simulink model "Adaptive_SMC"  (R2017b)
settings: Solver=ode45  StartTime=0.0  StopTime=20  RelTol=1e-3  EnableMultiTasking=on
settings Model: Creator=rushik  LastModifiedBy=thapa
settings SolverCC: MaxConsecutiveMinStep=5  ZeroCrossControl=EnableAll
settings DataIOCC: SaveOutput=off  SaveTime=off
settings OptimizationCC: LifeSpan=inf
settings DebuggingCC: SFUnexpectedBacktrackingDiag=warning  SFNoUnconditionalDefaultTransitionDiag=warning  SFExecutionAtInitializationDiag=none
settings ModelReferenceCC: ModelReferenceMinAlgLoopOccurrences=on
settings CodeAppCC: StateflowObjectComments=on
settings GRTTargetCC: TargetLangStandard=C89/C90 (ANSI)  CombineOutputUpdateFcns=off
settings ConfigComp: CovMetricSettings=dw  CovHtmlReporting=on  CovSaveCumulativeToWorkspaceVar=on  CovSaveSingleToWorkspaceVar=on  CovExternalEMLEnable=off

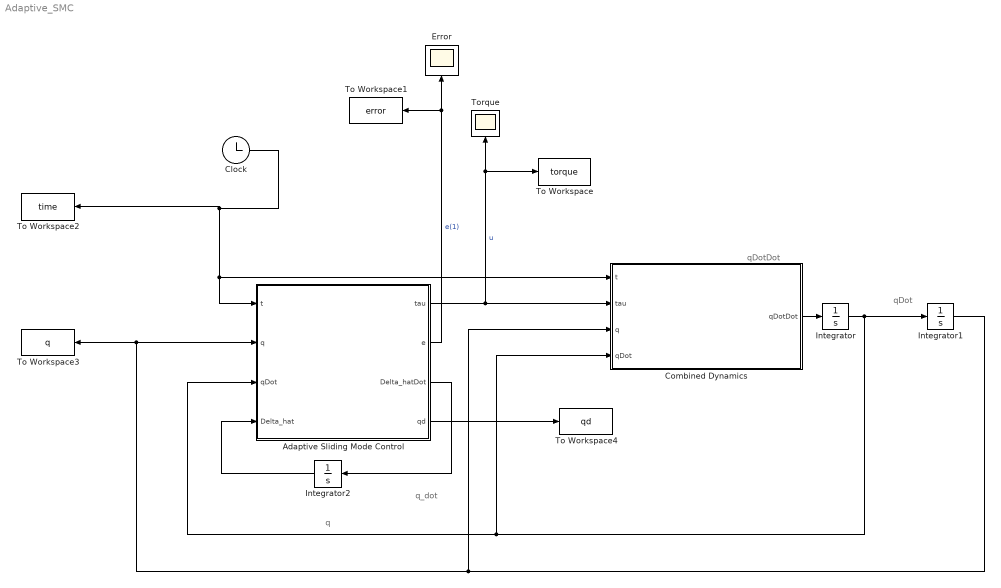
== system Adaptive_SMC ==
  note: q_dot
  note: q
  note: qDot
  note: qDotDot
  "Adaptive Sliding Mode Control " : MATLAB Function  TreatAsAtomicUnit=on
  Clock : Clock
      settings: Decimation=100
  "Combined Dynamics " : MATLAB Function  TreatAsAtomicUnit=on
  "Error " : Scope
  Integrator : Integrator  InitialCondition=[0;0;0;0;0;0;0;pi/2]  IgnoreLimit=on
  Integrator1 : Integrator  InitialCondition=[0;0;0;0;0;0;0;0]
  Integrator2 : Integrator  InitialCondition=[0;0;0;0;0;0;0;0]  IgnoreLimit=on
  To Workspace : ToWorkspace  VariableName=torque  SampleTime=-1
  To Workspace1 : ToWorkspace  VariableName=error  SampleTime=-1
  To Workspace2 : ToWorkspace  VariableName=time  SampleTime=-1
  To Workspace3 : ToWorkspace  VariableName=q  SampleTime=-1
  To Workspace4 : ToWorkspace  VariableName=qd  SampleTime=-1
  "Torque " : Scope
  wires:
  "Adaptive Sliding Mode Control "/1(tau) -> "Torque "/1, To Workspace/1, "Combined Dynamics "/2(tau)  "u"
  "Combined Dynamics "/1(qDotDot) -> Integrator/1
  Clock/1 -> "Adaptive Sliding Mode Control "/1(t), "Combined Dynamics "/1(t), To Workspace2/1
  "Adaptive Sliding Mode Control "/2(e) -> To Workspace1/1, "Error "/1  "e(1)"
  "Adaptive Sliding Mode Control "/3(Delta_hatDot) -> Integrator2/1
  Integrator2/1 -> "Adaptive Sliding Mode Control "/4(Delta_hat)
  Integrator/1 -> Integrator1/1, "Combined Dynamics "/4(qDot), "Adaptive Sliding Mode Control "/3(qDot)
  Integrator1/1 -> "Combined Dynamics "/3(q), To Workspace3/1, "Adaptive Sliding Mode Control "/2(q)
  "Adaptive Sliding Mode Control "/4(qd) -> To Workspace4/1

== matlab function Adaptive_SMC/Combined Dynamics  ==
  data: t input; tau input; qDotDot output; q input; qDot input
% Robot manipulator dynamics.
function qDotDot  = Aerial_Manipulator_dynamics(t, tau, q, qDot)

% q1 = q(1); q2 = q(2); % Joint angles
% q1_dot = q_dot(1); q2_dot = q_dot(2); % Joint angular velocities

x = q(1); 
y = q(2);
z = q(3);
phi = q(4);
theta = q(5);
psi = q(6); 
n1 = q(7);
n2 = q(8);

x_dot = qDot(1);
y_dot = qDot(2);
z_dot = qDot(3);
phi_dot = qDot(4);
theta_dot = qDot(5); 
psi_dot = qDot(6);
n1_dot = qDot(7);
n2_dot = qDot(8);

qd = [0 0 6 0 0 0 .5 .5]';
qdDot = [0 0 0 0 0 0 0 0]';
qdDotDot = [0 0 0 0 0 0 0 0]';

lamda = eye(8,8);
e = q - qd; 
eDot = qDot - qdDot;
s = eDot + lamda*e;
qrDot = qdDot-lamda*e;
qrDotDot = qdDotDot - lamda*eDot;

m_b = 2; 
Ixx = 1.24; 
Iyy = 1.24;
Izz = 2.48; 

m_1 = 0.049 ; 
Ix1 = 0.0011; 
Iy1 = Ix1; 
Iz1 = 0;
l1 = 0.015; 
l2 = 0.005;

Ix2 = 1.25/10000; 
Iy2 = Ix2; 
Iz2 = 0; 

m_2 = 0.05 ; 

p_b = [x y z]'; %postion of UAV with respect to inertial frame
p_b_dot = [x_dot y_dot z_dot]';
% An_b = [psi theta phi]'; %Euler angles used: yaw pitch roll 
% An_dot = [psi_dot theta_dot phi_dot]';
% n_b = [n1 n2]';  % joint angles 
n_dot = [n1_dot n2_dot]'; % joint angles rate 

T_b = [ 0, -sin(psi), cos(psi)*cos(theta); 
        0,  cos(psi), cos(theta)*sin(psi); 
        1,         0,         -sin(theta)];
    
R_b = [ cos(psi)*cos(theta), cos(psi)*sin(phi)*sin(theta) - cos(phi)*sin(psi), sin(phi)*sin(psi) + cos(phi)*cos(psi)*sin(theta); 
      cos(theta)*sin(psi), cos(phi)*cos(psi) + sin(phi)*sin(psi)*sin(theta),   cos(phi)*sin(psi)*sin(theta) - cos(psi)*sin(phi);
      -sin(theta),         cos(theta)*sin(phi),                              cos(phi)*cos(theta)];
 
Q = R_b'*T_b;

h1 = [1 0 0]'; 
P10 = [0 0 0.1]';
p1c = [0 0 l1/2]';

R01 = expm((hat(h1))*n1);

p1c_b = P10 + R01*p1c;    % in base frame 
p1c_i = p_b + R_b*p1c_b;  % in inertial frame

% position of center of link 2 
h2 = [0 1 0]';
p12 = [0 0 l1]';
p2T = [0 l2 0]';
p2c = [0 l2/2 0]';

R12 = expm((hat(h2))*n2);
R02 = R01*R12;

p2c_b = P10 + R01*p1c + R02*p2c;   % in base frame
p2c_i = p_b + R_b*p2c_b;  % in inertial frame

% position of end effector 

p2_b = P10 + R01*p12 + R02*p2T;   % in base frame
p2_i = p_b + R_b*p2_b;  % in inertial frame

Jw1c = [h1 zeros(3,1)];
Jv1c = [hat(h1)*p1c_b zeros(3,1)];
J1c = [Jw1c; Jv1c];
% Jacobian for link 2 center 
Jw2c = [h1 h2];
Jv2c = [hat(h1)*(R01*p12) hat(h2)*p2c_b];
J2c = [Jw2c; Jv2c];

% J2c = [h1 h2; hat(h1)*(R01*p12) hat(h2)*p2c_b];
% Jacobian for end effector 
JT = [h1 h2; hat(h1)*R01*p12 hat(h2)*p2_b];
JwT = JT(1:3,1:2);
JvT = JT(4:6,1:2);

% Kinetic Energy of UAV 
I_b = [Ixx 0 0;0 Iyy 0;0 0 Izz]';
I_1 = [Ix1 0 0;0 Iy1 0;0 0 Iz1]';
I_2 = [Ix2 0 0;0 Iy2 0;0 0 Iz2]';

% Inertia matrix B % Need to calculate the matrix 

M11 = (m_b + m_1 + m_2)*eye(3);

M22 = Q'*I_b*Q  +  m_1*T_b'*hat((R_b*p1c_b)')*hat(R_b*p1c_b)*T_b + Q'*R01*I_1*R01'*Q ...
        + m_2*T_b'*hat((R_b*p2c_b)')*hat(R_b*p2c_b)*T_b + Q'*R02*I_2*R02'*Q ;
    
M33 = m_1*(Jv1c)'*Jv1c + Jw1c'*R01*I_1*R01'*Jw1c ...
      + m_2*(Jv2c)'*Jv2c + Jw2c'*R02*I_2*R02'*Jw2c;
M12 = -(m_1*hat((R_b*p1c_b)')) -(m_2*hat((R_b*p2c_b)'));
M21 = M12';
M13 = m_1*R_b*Jv1c + m_2*R_b*Jv2c;
M31 = M13';
M23 = Q'*R01*I_1*R01'*Jw1c -m_1*T_b'*hat((R_b*p1c_b)')*R_b*Jv1c ...
      +Q'*R02*I_2*R02'*Jw2c -m_2*T_b'*hat((R_b*p2c_b)')*R_b*Jv2c ;
M32 = M23';

M1 = [M11,M12,M13];
M2 = [M21,M22,M23];
M3 = [M31,M32,M33];

M = [M1;M2;M3];
%  
C = C_Matrix_vars(2,0.049,0.05,1.24,1.24,2.48,0.0011,0.0011,0,0.000125,0.000125,0,0.015,0.005,q(1),q(2),q(3),q(4),q(5),q(6),q(7),q(8),qDot(1),qDot(2),qDot(3),qDot(4),qDot(5),qDot(6),qDot(7),qDot(8));

G1 = 0; 
G2 = 0; 
G3 = (49*m_1)/5 + (49*m_2)/5 + (49*m_b)/5; 
G4 = - (49*m_2*(cos(phi)*cos(theta)*((l1*sin(n1))/2 - (l2*cos(n1)*cos(n2))/2) + cos(theta)*sin(phi)*((l1*cos(n1))/2 + (l2*cos(n2)*sin(n1))/2)))/5 - (49*m_1*((l1*cos(n1)*cos(theta)*sin(phi))/2 + (l1*cos(phi)*cos(theta)*sin(n1))/2))/5;
G5 = (49*m_2*((l2*cos(theta)*sin(n2))/2 - cos(phi)*sin(theta)*((l1*cos(n1))/2 + (l2*cos(n2)*sin(n1))/2) + sin(phi)*sin(theta)*((l1*sin(n1))/2 - (l2*cos(n1)*cos(n2))/2)))/5 - (49*m_1*((l1*cos(n1)*cos(phi)*sin(theta))/2 - (l1*sin(n1)*sin(phi)*sin(theta))/2))/5;
G6 = 0; 
G7 = - (49*m_2*(cos(phi)*cos(theta)*((l1*sin(n1))/2 - (l2*cos(n1)*cos(n2))/2) + cos(theta)*sin(phi)*((l1*cos(n1))/2 + (l2*cos(n2)*sin(n1))/2)))/5 - (49*m_1*((l1*cos(n1)*cos(theta)*sin(phi))/2 + (l1*cos(phi)*cos(theta)*sin(n1))/2))/5;
G8 = -(49*m_2*((l2*cos(n1)*cos(theta)*sin(n2)*sin(phi))/2 - (l2*cos(n2)*sin(theta))/2 + (l2*cos(phi)*cos(theta)*sin(n1)*sin(n2))/2))/5; 

G = [G1;G2;G3;G4;G5;G6;G7;G8]; 

temp1 = -hat(R_b*p2_b)*T_b;
temp2 = R_b*JvT;

J_a = [eye(3,3)  , zeros(3,3),    zeros(3,2); 
       zeros(3,3), T_b       ,    zeros(3,2);
       eye(2,3)  , temp1(1:2,1:3),temp2(1:2,1:2)]; 
if t <10
    z_ext = (sin(pi/4*t));
    f_ext = [0 0 z_ext 0 0 0 0 0]';
    tau_ext = J_a'*f_ext;
    if z_ext < 0
       f_ext = [0 0 0 0 0 0 0 0]';
       tau_ext = J_a'*f_ext;
    end
else 
    f_ext = [0 0 0 0 0 0 0 0]';
    tau_ext = J_a'*f_ext;
end 

qDotDot = inv(M)*(tau + tau_ext -C*qDot -G);

== matlab function Adaptive_SMC/Adaptive Sliding Mode Control  ==
  data: t input; tau output; q input; qDot input; e output; Delta_hat input; Delta_hatDot output; qd output

function [tau, e, Delta_hatDot, qd]= Adaptive_SlidingMC(t,q, qDot, Delta_hat)

qd = [0 0 6 0 0 0 .5 .5]';
qdDot = [0 0 0 0 0 0 0 0]';
qdDotDot = [0 0 0 0 0 0 0 0]';

lamda = 2*eye(8,8);
e = q - qd; 
eDot = qDot - qdDot;
s = eDot - lamda*e;
qrDot = qdDot-lamda*e;
qrDotDot = qdDotDot - lamda*eDot;

M_hat = eye(8,8);
C_hat = eye(8,8);
G_hat = [0 0 10 0 0 0 0 0]';
A = eye(8,8);
K = eye(8,8);

x = q(1); 
y = q(2);
z = q(3);
phi = q(4);
theta = q(5);
psi = q(6); 
n1 = q(7);
n2 = q(8);

x_dot = qDot(1);
y_dot = qDot(2);
z_dot = qDot(3);
phi_dot = qDot(4);
theta_dot = qDot(5); 
psi_dot = qDot(6);
n1_dot = qDot(7);
n2_dot = qDot(8);

lamda = eye(8,8);
e = q - qd; 
eDot = qDot - qdDot;
s = eDot + lamda*e;
qrDot = qdDot-lamda*e;
qrDotDot = qdDotDot - lamda*eDot;

m_b = 2; 
Ixx = 1.24; 
Iyy = 1.24;
Izz = 2.48; 

m_1 = 0.049 ; 
Ix1 = 0.0011; 
Iy1 = Ix1; 
Iz1 = 0;
l1 = 0.015; 
l2 = 0.005;

Ix2 = 1.25/10000; 
Iy2 = Ix2; 
Iz2 = 0; 

m_2 = 0.05 ; 

p_b = [x y z]'; %postion of UAV with respect to inertial frame
p_b_dot = [x_dot y_dot z_dot]';
% An_b = [psi theta phi]'; %Euler angles used: yaw pitch roll 
% An_dot = [psi_dot theta_dot phi_dot]';
% n_b = [n1 n2]';  % joint angles 
n_dot = [n1_dot n2_dot]'; % joint angles rate 

T_b = [ 0, -sin(psi), cos(psi)*cos(theta); 
        0,  cos(psi), cos(theta)*sin(psi); 
        1,         0,         -sin(theta)];
    
R_b = [ cos(psi)*cos(theta), cos(psi)*sin(phi)*sin(theta) - cos(phi)*sin(psi), sin(phi)*sin(psi) + cos(phi)*cos(psi)*sin(theta); 
      cos(theta)*sin(psi), cos(phi)*cos(psi) + sin(phi)*sin(psi)*sin(theta),   cos(phi)*sin(psi)*sin(theta) - cos(psi)*sin(phi);
      -sin(theta),         cos(theta)*sin(phi),                              cos(phi)*cos(theta)];
  
Q = R_b'*T_b;

h1 = [1 0 0]'; 
P10 = [0 0 0.1]';
p1c = [0 0 l1/2]';

R01 = expm((hat(h1))*n1);

p1c_b = P10 + R01*p1c;    % in base frame 
p1c_i = p_b + R_b*p1c_b;  % in inertial frame

% position of center of link 2 
h2 = [0 1 0]';
p12 = [0 0 l1]';
p2T = [0 l2 0]';
p2c = [0 l2/2 0]';

R12 = expm((hat(h2))*n2);
R02 = R01*R12;

p2c_b = P10 + R01*p1c + R02*p2c;   % in base frame
p2c_i = p_b + R_b*p2c_b;  % in inertial frame

% position of end effector 

p2_b = P10 + R01*p12 + R02*p2T;   % in base frame
p2_i = p_b + R_b*p2_b;  % in inertial frame

Jw1c = [h1 zeros(3,1)];
Jv1c = [hat(h1)*p1c_b zeros(3,1)];
J1c = [Jw1c; Jv1c];
% Jacobian for link 2 center 
Jw2c = [h1 h2];
Jv2c = [hat(h1)*(R01*p12) hat(h2)*p2c_b];
J2c = [Jw2c; Jv2c];

% J2c = [h1 h2; hat(h1)*(R01*p12) hat(h2)*p2c_b];
% Jacobian for end effector 
JT = [h1 h2; hat(h1)*R01*p12 hat(h2)*p2_b];
JwT = JT(1:3,1:2);
JvT = JT(4:6,1:2);

% Dynamic Model of Aerial Manipulator 
% Kinetic Energy of UAV 
I_b = [Ixx 0 0;0 Iyy 0;0 0 Izz]';
I_1 = [Ix1 0 0;0 Iy1 0;0 0 Iz1]';
I_2 = [Ix2 0 0;0 Iy2 0;0 0 Iz2]';

% Inertia matrix B % Need to calculate the matrix 

M11 = (m_b + m_1 + m_2)*eye(3);

M22 = Q'*I_b*Q  +  m_1*T_b'*hat((R_b*p1c_b)')*hat(R_b*p1c_b)*T_b + Q'*R01*I_1*R01'*Q ...
        + m_2*T_b'*hat((R_b*p2c_b)')*hat(R_b*p2c_b)*T_b + Q'*R02*I_2*R02'*Q ;
    
M33 = m_1*(Jv1c)'*Jv1c + Jw1c'*R01*I_1*R01'*Jw1c ...
      + m_2*(Jv2c)'*Jv2c + Jw2c'*R02*I_2*R02'*Jw2c;
M12 = -(m_1*hat((R_b*p1c_b)')) -(m_2*hat((R_b*p2c_b)'));
M21 = M12';
M13 = m_1*R_b*Jv1c + m_2*R_b*Jv2c;
M31 = M13';
M23 = Q'*R01*I_1*R01'*Jw1c -m_1*T_b'*hat((R_b*p1c_b)')*R_b*Jv1c ...
      +Q'*R02*I_2*R02'*Jw2c -m_2*T_b'*hat((R_b*p2c_b)')*R_b*Jv2c ;
M32 = M23';

M1 = [M11,M12,M13];
M2 = [M21,M22,M23];
M3 = [M31,M32,M33];

M = [M1;M2;M3];

%  
C = C_Matrix_vars(2,0.049,0.05,1.24,1.24,2.48,0.0011,0.0011,0,0.000125,...
    0.000125,0,0.015,0.005,q(1),q(2),q(3),q(4),q(5),q(6),q(7),q(8),...
    qDot(1),qDot(2),qDot(3),qDot(4),qDot(5),qDot(6),qDot(7),qDot(8));

G1 = 0; 
G2 = 0; 
G3 = (49*m_1)/5 + (49*m_2)/5 + (49*m_b)/5; 
G4 = - (49*m_2*(cos(phi)*cos(theta)*((l1*sin(n1))/2 - (l2*cos(n1)*cos(n2))/2)...
    + cos(theta)*sin(phi)*((l1*cos(n1))/2 + (l2*cos(n2)*sin(n1))/2)))/5 - ...
    (49*m_1*((l1*cos(n1)*cos(theta)*sin(phi))/2 + ...
    (l1*cos(phi)*cos(theta)*sin(n1))/2))/5;
G5 = (49*m_2*((l2*cos(theta)*sin(n2))/2 - cos(phi)*sin(theta)*((l1*cos(n1))/2 +...
    (l2*cos(n2)*sin(n1))/2) + sin(phi)*sin(theta)*((l1*sin(n1))/2 -...
    (l2*cos(n1)*cos(n2))/2)))/5 - (49*m_1*((l1*cos(n1)*cos(phi)*sin(theta))/2 - ...
    (l1*sin(n1)*sin(phi)*sin(theta))/2))/5;
G6 = 0; 
G7 = - (49*m_2*(cos(phi)*cos(theta)*((l1*sin(n1))/2 - (l2*cos(n1)*cos(n2))/2) +...
    cos(theta)*sin(phi)*((l1*cos(n1))/2 + (l2*cos(n2)*sin(n1))/2)))/5 - ...
    (49*m_1*((l1*cos(n1)*cos(theta)*sin(phi))/2 + (l1*cos(phi)*cos(theta)*sin(n1))/2))/5;
G8 = -(49*m_2*((l2*cos(n1)*cos(theta)*sin(n2)*sin(phi))/2 - (l2*cos(n2)*sin(theta))/2 + ...
    (l2*cos(phi)*cos(theta)*sin(n1)*sin(n2))/2))/5; 

G = [G1;G2;G3;G4;G5;G6;G7;G8];

M_telta = M_hat - M; 
C_telta = C_hat - C;
G_telta = G_hat - G;

Delta = -M_telta*qrDotDot - C_telta*qrDot - G_telta;

Detla_telta = Delta_hat - Delta; 
Kp = 80*eye(8,8);
Kv = 10*eye(8,8);
K = 8*eye(8,8);
A = 10*eye(8,8);

% tau = M_hat*qrDotDot + C_hat*qrDot + G_hat + Delta_hat - Kv*eDot- Kp*e;
tau = M_hat*qrDotDot + C_hat*qrDot + G_hat + Delta_hat - A*s - K*sign(s); 
K_g = 10*eye(8,8);

Delta_hatDot = -K_g*s;
